simulink model "FuncionTransferenciaProy"  (R2024a)
settings: Solver=VariableStepAuto  StartTime=0.0  StopTime=8  RelTol=1e-3
libraries: simulink x3
settings Model: Creator=danid  LastModifiedBy=danid

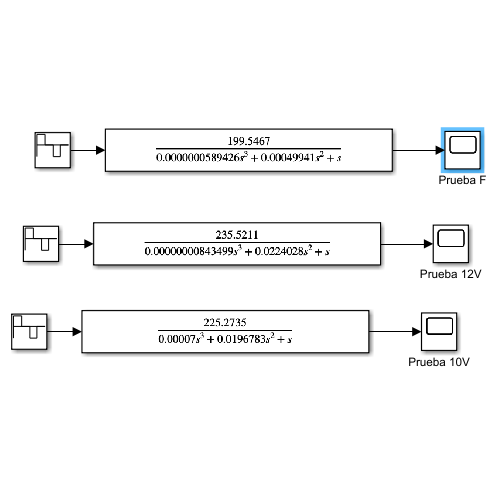
[thumbnail: Simulink's stored preview of the top-level diagram]
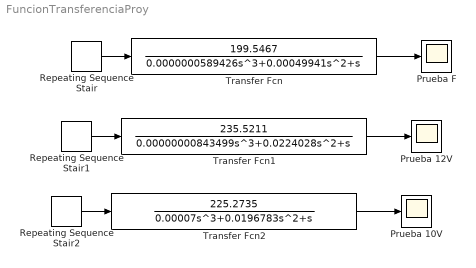
== system FuncionTransferenciaProy ==
  Prueba 10V : Scope
  Prueba 12V : Scope
  Prueba F : Scope
  Repeating Sequence Stair : simulink/Sources/Repeating Sequence Stair  OutValues=[10 0 -10 0].'  tsamp=1  OutMin=[]  OutMax=[]  OutDataTypeStr=double  OutputDataTypeScalingMode=double  OutDataType=fixdt(0,8)  ConRadixGroup=Best Precision: Vector-wise  OutScaling=2^-12
  Repeating Sequence Stair1 : simulink/Sources/Repeating Sequence Stair  OutValues=[12 0 -12 0].'  tsamp=1  OutMin=[]  OutMax=[]  OutDataTypeStr=double  OutputDataTypeScalingMode=double  OutDataType=fixdt(0,8)  ConRadixGroup=Best Precision: Vector-wise  OutScaling=2^-12
  Repeating Sequence Stair2 : simulink/Sources/Repeating Sequence Stair  OutValues=[10 0 -10 0].'  tsamp=1  OutMin=[]  OutMax=[]  OutDataTypeStr=double  OutputDataTypeScalingMode=double  OutDataType=fixdt(0,8)  ConRadixGroup=Best Precision: Vector-wise  OutScaling=2^-12
  Transfer Fcn : TransferFcn  Numerator=[199.5467]  Denominator=[0.0000000589426 0.00049941 1 0]
  Transfer Fcn1 : TransferFcn  Numerator=[235.5211]  Denominator=[0.00000000843499 0.0224028 1 0]
  Transfer Fcn2 : TransferFcn  Numerator=[225.2735]  Denominator=[0.00007 0.0196783 1 0]
  wires:
  Repeating Sequence Stair/1 -> Transfer Fcn/1
  Transfer Fcn/1 -> Prueba F/1
  Transfer Fcn1/1 -> Prueba 12V/1
  Repeating Sequence Stair1/1 -> Transfer Fcn1/1
  Transfer Fcn2/1 -> Prueba 10V/1
  Repeating Sequence Stair2/1 -> Transfer Fcn2/1
